simulink model "udpdron"  (R2025a)
settings: Solver=FixedStepAuto  StartTime=0.0  StopTime=inf  FixedStep=0.001  RelTol=1e-3  EnableMultiTasking=on
libraries: etargetslib x9, dspnetwork x9, px4Sensorslib x2, px4Peripheralslib x1
settings Model: PacingRate=0.790000  ExtModeTrigDuration=10  Creator=The MathWorks, Inc.  LastModifiedBy=aero
settings SolverCC: AlgebraicLoopSolver=TrustRegion  PositivePriorityOrder=on  AutoInsertRateTranBlk=on  MaxZcPerStep=1.0
settings OptimizationCC: EnhancedBackFolding=on  PassReuseOutputArgsAs=Individual arguments  MaxStackSize=64  OptimizeBlockOrder=speed  DifferentSizesBufferReuse=on  OptimizationCustomize=off  EfficientTunableParamExpr=on
settings DebuggingCC: ParameterPrecisionLossMsg=none  ParameterTunabilityLossMsg=error  UnconnectedInputMsg=warning  UnconnectedOutputMsg=warning  UnconnectedLineMsg=warning  SubsystemReferenceDiagnosticForUnitTest=warning  ArithmeticOperatorsInVariantConditions=warning
settings HardwareCC: ProdBitPerPointer=32.0  ProdBitPerSizeT=32.0  ProdBitPerPtrDiffT=32.0  ProdLargestAtomicInteger=Long  ProdLargestAtomicFloat=Double  ProdWordSize=32.0  ProdLongLongMode=on  ProdHWDeviceType=ARM Compatible->ARM Cortex
settings ModelReferenceCC: EnableRefExpFcnMdlSchedulingChecks=on
settings SFSimCC: MATLABDynamicMemAlloc=off  SimTargetLang=C++  SimDLTargetLibrary=mkl-dnn
settings RTWCC: SystemTargetFile=ert.tlc  HardwareBoard=PX4 Pixhawk 6c  TLCOptions="-aInlineSetEventsForThisBaseRateFcn=TLC_FALSE -aSuppressMultiTaskScheduler=TLC_FALSE  -aRateBasedStepFcn=0"  TemplateMakefile=ert_default_tmf  GenerateReport=on  Toolchain=GNU Tools for PX4 Autopilots  IncludeHyperlinkInReport=on  LaunchReport=on  TargetLang=C++  GenerateTraceInfo=on  GenerateTraceReport=on  GenerateTraceReportSl=on  GenerateTraceReportSf=on  GenerateTraceReportEml=on  GPUComputeCapability=3.5  DLArmComputeVersion=19.05  Description=Embedded Coder
settings CodeAppCC: ForceParamTrailComments=on  IgnoreCustomStorageClasses=off  OperatorAnnotations=on  SimulinkDataObjDesc=on  SFDataObjDesc=on  InsertBlockDesc=on
settings ERTTargetCC: ExtModeTransport=3.0  ExtModeStaticAllocSize=1024.0  InlinedParameterPlacement=Hierarchical

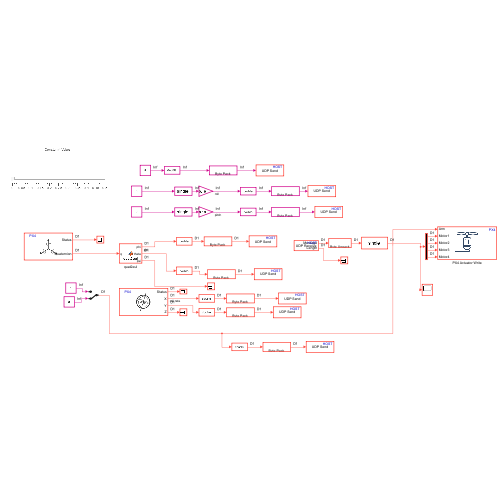
[thumbnail: Simulink's stored preview of the top-level diagram]
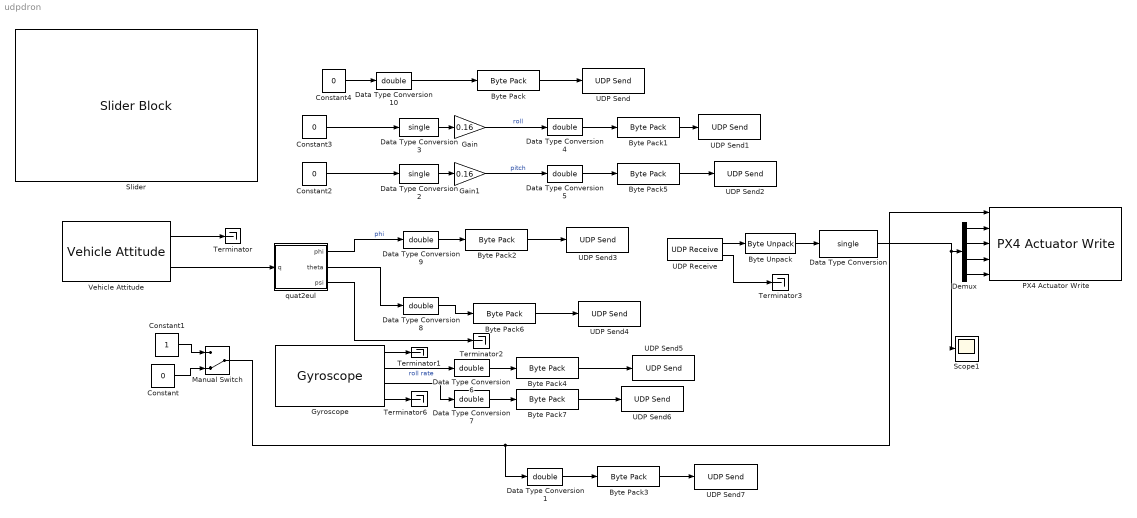
== system udpdron ==
  Byte Pack{,1..7} (8 alike) : etargetslib/Byte Pack  datatypes={'double'}  byteAlign=8
  Byte Unpack : etargetslib/Byte Unpack  dimensions={[4]}  datatypes={'double'}  byteAlign=8
      settings: LibrarySourceBlock=embeddedtargetslib/Host Communication/Byte Unpack
  Constant : Constant  Value=0  OutDataTypeStr=boolean
  Constant1 : Constant  OutDataTypeStr=boolean
  Constant2 : Constant  Value=0
  Constant3 : Constant  Value=0
  Constant4 : Constant  Value=0
  Data Type Conversion : DataTypeConversion  OutDataTypeStr=single  SaturateOnIntegerOverflow=off  RndMeth=Floor
  Data Type Conversion{1,4..10} (8 alike) : DataTypeConversion  OutDataTypeStr=double  SaturateOnIntegerOverflow=off  RndMeth=Floor
  Data Type Conversion2 : DataTypeConversion  OutDataTypeStr=single  SaturateOnIntegerOverflow=off  RndMeth=Floor
  Data Type Conversion3 : DataTypeConversion  OutDataTypeStr=single  SaturateOnIntegerOverflow=off  RndMeth=Floor
  Demux : Demux
  Gain : Gain  Gain=0.16
  Gain1 : Gain  Gain=0.16
  Gyroscope : px4Sensorslib/Gyroscope  uorbTimeStamp=off  BlockingMode=off  BlockTimeout=1e-3  sampleTime=0.001
  Manual Switch : ManualSwitch  CurrentSetting=0
  PX4 Actuator Write : px4Peripheralslib/PX4 Actuator Write  Motor1Enable=on  Motor2Enable=on  Motor3Enable=on  Motor4Enable=on  Motor5Enable=off  Motor6Enable=off  Motor7Enable=off  Motor8Enable=off  Motor9Enable=off  Motor10Enable=off  Motor11Enable=off  Motor12Enable=off  IsMotorArray=off  Servo1Enable=off  Servo2Enable=off  Servo3Enable=off  Servo4Enable=off  Servo5Enable=off  Servo6Enable=off  Servo7Enable=off  Servo8Enable=off  IsServoArray=off
  Scope1 : Scope
      settings: ActiveDisplayYMinimum=0.37234214547850747  ActiveDisplayYMaximum=0.42208466280379647  DataLoggingVariableName=ScopeData3
  Slider : SliderBlock  ScaleMax=0.5
  Terminator{,1..3,6} (5 alike) : Terminator
  UDP Receive : dspnetwork/UDP Receive  localURL='0.0.0.0'  localPort=25008  remoteURL='0.0.0.0'  remotePort=-1  recvBufferSize=8192  dims=32  signalDatatype=uint8  isComplex=off  isVarSize=off  showBlockingTime=on  blockingTime=0  sampletime=0.001  blockPlatform=HOST
      settings: LibrarySourceBlock=embeddedtargetslib/Host Communication/UDP Receive
  UDP Send : dspnetwork/UDP Send  remoteURL='127.0.0.1'  remotePort=25000  localURL='0.0.0.0'  localPortSource=Automatically determine  localPort=-1  sendBufferSize=8192  sampletime=-1  blockPlatform=HOST  separateLengthPort=0
      settings: LibrarySourceBlock=embeddedtargetslib/Host Communication/UDP Send
  UDP Send1 : dspnetwork/UDP Send  remoteURL='127.0.0.1'  remotePort=25001  localURL='0.0.0.0'  localPortSource=Automatically determine  localPort=-1  sendBufferSize=8192  sampletime=-1  blockPlatform=HOST  separateLengthPort=0
      settings: LibrarySourceBlock=embeddedtargetslib/Host Communication/UDP Send
  UDP Send2 : dspnetwork/UDP Send  remoteURL='127.0.0.1'  remotePort=25002  localURL='0.0.0.0'  localPortSource=Automatically determine  localPort=-1  sendBufferSize=8192  sampletime=-1  blockPlatform=HOST  separateLengthPort=0
      settings: LibrarySourceBlock=embeddedtargetslib/Host Communication/UDP Send
  UDP Send3 : dspnetwork/UDP Send  remoteURL='127.0.0.1'  remotePort=25003  localURL='0.0.0.0'  localPortSource=Automatically determine  localPort=-1  sendBufferSize=8192  sampletime=-1  blockPlatform=HOST  separateLengthPort=0
      settings: LibrarySourceBlock=embeddedtargetslib/Host Communication/UDP Send
  UDP Send4 : dspnetwork/UDP Send  remoteURL='127.0.0.1'  remotePort=25004  localURL='0.0.0.0'  localPortSource=Automatically determine  localPort=-1  sendBufferSize=8192  sampletime=-1  blockPlatform=HOST  separateLengthPort=0
      settings: LibrarySourceBlock=embeddedtargetslib/Host Communication/UDP Send
  UDP Send5 : dspnetwork/UDP Send  remoteURL='127.0.0.1'  remotePort=25005  localURL='0.0.0.0'  localPortSource=Automatically determine  localPort=-1  sendBufferSize=8192  sampletime=-1  blockPlatform=HOST  separateLengthPort=0
      settings: LibrarySourceBlock=embeddedtargetslib/Host Communication/UDP Send
  UDP Send6 : dspnetwork/UDP Send  remoteURL='127.0.0.1'  remotePort=25006  localURL='0.0.0.0'  localPortSource=Automatically determine  localPort=-1  sendBufferSize=8192  sampletime=-1  blockPlatform=HOST  separateLengthPort=0
      settings: LibrarySourceBlock=embeddedtargetslib/Host Communication/UDP Send
  UDP Send7 : dspnetwork/UDP Send  remoteURL='127.0.0.1'  remotePort=25007  localURL='0.0.0.0'  localPortSource=Automatically determine  localPort=-1  sendBufferSize=8192  sampletime=-1  blockPlatform=HOST  separateLengthPort=0
      settings: LibrarySourceBlock=embeddedtargetslib/Host Communication/UDP Send
  Vehicle Attitude : px4Sensorslib/Vehicle Attitude  rollRate=off  pitchRate=off  yawRate=off  quaternion=on  uorbTimeStamp=off  BlockingMode=off  BlockTimeout=0.001  sampleTime=0.001
  quat2eul : MATLAB Function  TreatAsAtomicUnit=on
  wires:
  Manual Switch/1 -> Data Type Conversion1/1, PX4 Actuator Write/1
  Vehicle Attitude/1 -> Terminator/1
  Gyroscope/1 -> Terminator1/1
  Gain/1 -> Data Type Conversion4/1  "roll"
  Byte Unpack/1 -> Data Type Conversion/1
  Demux/1 -> PX4 Actuator Write/2
  Demux/2 -> PX4 Actuator Write/3
  Demux/3 -> PX4 Actuator Write/4
  Demux/4 -> PX4 Actuator Write/5
  Constant/1 -> Manual Switch/2
  Constant1/1 -> Manual Switch/1
  Gyroscope/2 -> Data Type Conversion6/1  "roll rate"
  Gyroscope/4 -> Terminator6/1
  Gyroscope/3 -> Data Type Conversion7/1
  Gain1/1 -> Data Type Conversion5/1  "pitch"
  Data Type Conversion3/1 -> Gain/1
  Data Type Conversion2/1 -> Gain1/1
  Constant2/1 -> Data Type Conversion2/1
  Constant3/1 -> Data Type Conversion3/1
  Vehicle Attitude/2 -> quat2eul/1(q)
  quat2eul/2(theta) -> Data Type Conversion8/1
  quat2eul/1(phi) -> Data Type Conversion9/1  "phi"
  quat2eul/3(psi) -> Terminator2/1
  Constant4/1 -> Data Type Conversion10/1
  Data Type Conversion1/1 -> Byte Pack3/1
  Data Type Conversion4/1 -> Byte Pack1/1
  Data Type Conversion5/1 -> Byte Pack5/1
  Data Type Conversion6/1 -> Byte Pack4/1
  Data Type Conversion8/1 -> Byte Pack6/1
  Data Type Conversion9/1 -> Byte Pack2/1
  Data Type Conversion10/1 -> Byte Pack/1
  Data Type Conversion7/1 -> Byte Pack7/1
  UDP Receive/1 -> Byte Unpack/1
  UDP Receive/2 -> Terminator3/1
  Byte Pack/1 -> UDP Send/1
  Byte Pack1/1 -> UDP Send1/1
  Byte Pack5/1 -> UDP Send2/1
  Byte Pack2/1 -> UDP Send3/1
  Byte Pack6/1 -> UDP Send4/1
  Byte Pack4/1 -> UDP Send5/1
  Byte Pack7/1 -> UDP Send6/1
  Byte Pack3/1 -> UDP Send7/1
  Data Type Conversion/1 -> Scope1/1, Demux/1

== matlab function udpdron/quat2eul ==
  data: q input; phi output; theta output; psi output
function [phi,theta,psi] = quat2eul(q)

% Quaternion conversion to Euler angles based on the PX4 Firmware v1.10.2
% release.

phi = atan2(2*(q(1)*q(2) + q(3)* q(4)), q(1)^2 - q(2)^2 - q(3)^2 + q(4)^2);
theta = asin(-2*(q(2)*q(4) - q(1)*q(3)));
psi = atan2(2*(q(2)*q(3) + q(1)* q(4)), q(1)^2 + q(2)^2 - q(3)^2 - q(4)^2);
end
